simulink model "momentum_unload_test"  (R2016b)
settings: Solver=VariableStepAuto  StartTime=0.0  StopTime=5400  MinStep=0.001  RelTol=1e-3
libraries: dynamics_lib x1, environment_lib x1, momentum_dump_lib_test x1, pd_control_lib x1, RW_assembly_simple_lib x1, command_processing x1, actuators_lib x1
settings Model: Creator=taylorreynolds  LastModifiedBy=evich

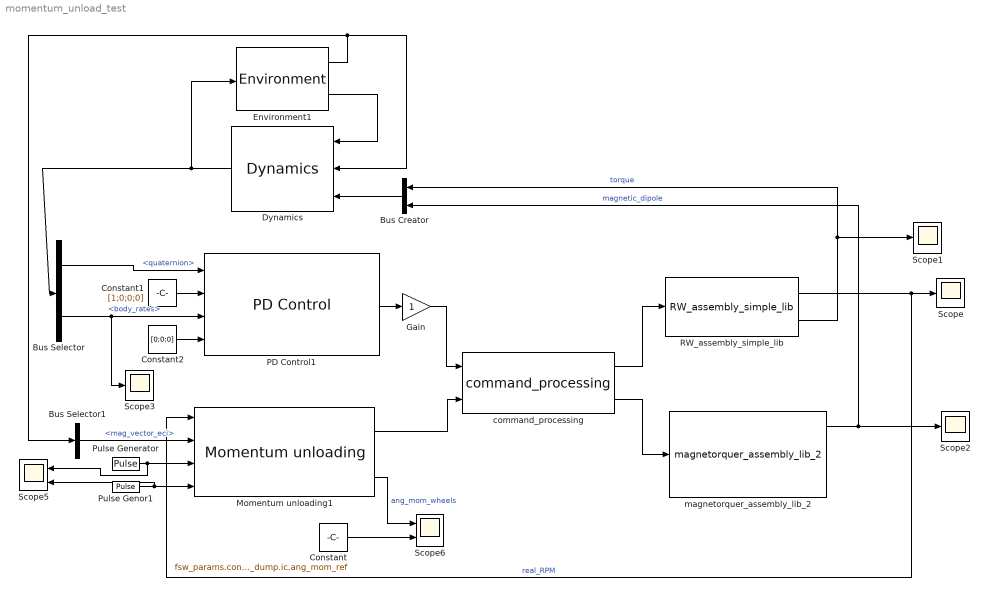
== system momentum_unload_test ==
  Bus Creator : BusCreator  Inputs=2
  Bus Selector : BusSelector  OutputSignals=quaternion,body_rates
  Bus Selector1 : BusSelector  OutputSignals=mag_vector_eci
  Constant : Constant  Value=fsw_params.control.p_dump.ic.ang_mom_ref
  Constant1 : Constant  Value=[1;0;0;0]
  Constant2 : Constant  Value=[0;0;0]
  Dynamics : dynamics_lib/Dynamics
  Environment1 : environment_lib/Environment
  Gain : Gain
  Momentum unloading1 : momentum_dump_lib_test/Momentum unloading
  PD Control1 : pd_control_lib/PD Control
  Pulse Generator : DiscretePulseGenerator  PulseType=Time based  Period=fsw_params.actuators.ppt.sync_pulse  PulseWidth=fsw_params.actuators.ppt.t_charge_pct
  Pulse Genor1 : DiscretePulseGenerator  PulseType=Time based  Period=10  PulseWidth=sim_params.sensors.magnetometer.valid_pct
  RW_assembly_simple_lib : RW_assembly_simple_lib/RW_assembly_simple_lib  natural_frequency=100  damping_ratio=1  max_rate=100
  Scope{,1..3} (4 alike) : Scope
  Scope5 : Scope  NumInputPorts=2
  Scope6 : Scope  NumInputPorts=2
  command_processing : command_processing/command_processing
  magnetorquer_assembly_lib_2 : actuators_lib/Actuators/magnetorquer_assembly_lib_2
  wires:
  Environment1/2 -> Dynamics/1
  Environment1/1 -> Dynamics/2, Bus Selector1/1
  Dynamics/1 -> Environment1/1, Bus Selector/1
  Bus Selector/2 -> Scope3/1, PD Control1/3  "<body_rates>"
  Bus Selector/1 -> PD Control1/1  "<quaternion>"
  Bus Creator/1 -> Dynamics/3
  magnetorquer_assembly_lib_2/1 -> Scope2/1, Bus Creator/2  "magnetic_dipole"
  RW_assembly_simple_lib/2 -> Scope1/1, Bus Creator/1  "torque"
  RW_assembly_simple_lib/1 -> Momentum unloading1/1, Scope/1  "real_RPM"
  Momentum unloading1/1 -> command_processing/2
  Bus Selector1/1 -> Momentum unloading1/2  "<mag_vector_eci>"
  Pulse Generator/1 -> Momentum unloading1/3, Scope5/1
  Pulse Genor1/1 -> Momentum unloading1/4, Scope5/2
  Momentum unloading1/2 -> Scope6/1  "ang_mom_wheels"
  Constant1/1 -> PD Control1/2
  Constant2/1 -> PD Control1/4
  Constant/1 -> Scope6/2
  PD Control1/1 -> Gain/1
  Gain/1 -> command_processing/1
  command_processing/1 -> RW_assembly_simple_lib/1
  command_processing/2 -> magnetorquer_assembly_lib_2/1
